simulink model "sm_car"  (R2026a)
settings: Solver=ode23t  StopTime=100  MaxStep=0.4  AbsTol=1e-3  EnableMultiTasking=on
PreLoadFcn:
  | % Due to usability issue in Repeating Sequence block
  | warning('off','Simulink:Masking:Invalid');
  | 
  | % Eliminate unnecessary warnings in inactive variants
  | % Warnings generated only if you click through inactive variant
  | warning('off','MATLAB:nonExistentField');
  | warning('off','Simulink:Parameters:BlkParamUndefined');
PostLoadFcn:
  | warning('off','sm:sli:setup:compile:LocalSolverNotSupported')
  | %sm_car_config_maneuver(bdroot,'WOT Braking');
  | sm_car_config_vehicle(bdroot,'false');
  | sm_car_config_logging(bdroot);
InitFcn:
  | sm_car_config_camera;
  | Vehicle = sm_car_vehcfg_checkConfig(Vehicle);
  | sm_car_check_tire_model(bdroot);
StartFcn:
  | tic;
StopFcn:
  | Elapsed_Sim_Time = toc;
  | % disp(['Elapsed Sim Time = ' num2str(Elapsed_Sim_Time)]);
undefined symbols (not defined in the file): Camera, Control, Driver, Maneuver, Pedal, Scene, Soft, Stiff, Visual, X, xy_data_car_side, Y, Z
libraries: sm_lib x207, simulink x21, nesl_utility x6, simulink_extras x4, slpidlib x1
(part 5 of 13)

== system sm_car/Driver/Closed Loop/Override ==
  "dist " : Inport
  "Obs " : Inport  Port=2
  None : Subsystem  VariantControl=None  mask(No Driver Override){override=Scene.Mallory_Park_Obstacle.Override}
      mask prompts: override "Override parameters (structure)"
      mask help: Driver commands are not overridden, regardless of inputs to subsystem.
  " Ovr" : Outport  VectorParamsAs1DForOutWhenUnconnected=off

== system sm_car/Driver/Closed Loop/Scopes ==
  <vx> : Inport
  Ref : Inport  Port=2
  CurPose : Inport  Port=3
  DrvBus : Inport  Port=4
  Bus Selector : BusSelector  OutputSignals=vTarget
  Bus Selector1 : BusSelector  OutputSignals=aSteerWheel,rAccelPedal,rBrakePedal
  Compare vx to Target : Scope  NumInputPorts=2
      settings: ActiveDisplayYMinimum=-4.79181  ActiveDisplayYMaximum=0.54534
  RefPose : Scope
      settings: ActiveDisplayYMinimum=-598.75829  ActiveDisplayYMaximum=469.37365
  Scope1 : Scope  NumInputPorts=3
      settings: ActiveDisplayYMinimum=-1.19495  ActiveDisplayYMaximum=0.13277  DataLoggingVariableName=ScopeData2
  wires:
  DrvBus/1 -> Bus Selector1/1
  Bus Selector1/1 -> Scope1/1  "<aSteerWheel>"
  Bus Selector1/2 -> Scope1/2  "<rAccelPedal>"
  <vx>/1 -> Compare vx to Target/1
  Bus Selector1/3 -> Scope1/3  "<rBrakePedal>"
  CurPose/1 -> RefPose/1
  Bus Selector/1 -> Compare vx to Target/2  "<vTarget>"
  Ref/1 -> Bus Selector/1

== system sm_car/Driver/Open Loop/Open Loop ==
  Bus Creator : BusCreator  Inputs=7
  Bus Creator5 : BusCreator  Inputs=4
  Constant : Constant  Value=10000
  Constant{1..6} (6 alike) : Constant  Value=0
  Input Sequence Accel Pedal : simulink/Sources/Repeating Sequence  rep_seq_t=Maneuver.Accel.t.Value  rep_seq_y=Maneuver.Accel.rPedal.Value
  Input Sequence Brake Pedal : simulink/Sources/Repeating Sequence  rep_seq_t=Maneuver.Brake.t.Value  rep_seq_y=Maneuver.Brake.rPedal.Value
  "Input Sequence Steering Wheel " : simulink/Sources/Repeating Sequence  rep_seq_t=Maneuver.Steer.t.Value  rep_seq_y=Maneuver.Steer.aWheel.Value
  DrvBus : Outport  VectorParamsAs1DForOutWhenUnconnected=off
  wires:
  Constant6/1 -> Bus Creator/7  "nLap"
  Constant/1 -> Bus Creator/1  "dist"
  Bus Creator/1 -> Bus Creator5/1  "Reference"
  Constant4/1 -> Bus Creator/5  "vTarget"
  Constant3/1 -> Bus Creator/4  "ayaw"
  Constant2/1 -> Bus Creator/3  "y"
  Constant5/1 -> Bus Creator/6  "latdev"
  Constant1/1 -> Bus Creator/2  "x"
  Input Sequence Accel Pedal/1 -> Bus Creator5/3  "rAccelPedal"
  "Input Sequence Steering Wheel "/1 -> Bus Creator5/2  "aSteerWheel"
  Input Sequence Brake Pedal/1 -> Bus Creator5/4  "rBrakePedal"
  Bus Creator5/1 -> DrvBus/1  "DrvBus"

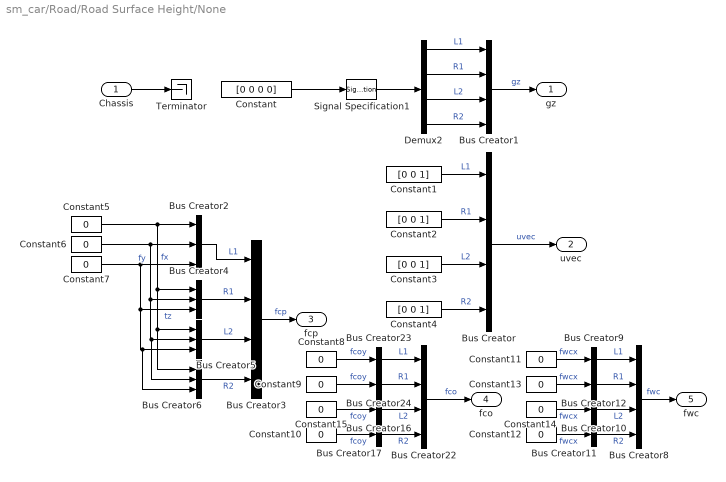
== system sm_car/Road/Road Surface Height/None ==
  Chassis : Inport
  Bus Creator{,1,3,8,22} (5 alike) : BusCreator  Inputs=4
  Bus Creator{9..12,16..17,23..24} (8 alike) : BusCreator  Inputs=1
  Bus Creator{2,4..6} (4 alike) : BusCreator  Inputs=3
  Constant : Constant  Value=[0 0 0 0]
  Constant{1..4} (4 alike) : Constant  Value=[0 0 1]
  Constant{5..15} (11 alike) : Constant  Value=0
  Demux2 : Demux
  Signal Specification1 : SignalSpecification  Unit=m
  Terminator : Terminator
  gz : Outport  VectorParamsAs1DForOutWhenUnconnected=off
  uvec : Outport  Port=2  VectorParamsAs1DForOutWhenUnconnected=off
  fcp : Outport  Port=3  VectorParamsAs1DForOutWhenUnconnected=off
  fco : Outport  Port=4  VectorParamsAs1DForOutWhenUnconnected=off
  fwc : Outport  Port=5  VectorParamsAs1DForOutWhenUnconnected=off
  wires:
  Bus Creator24/1 -> Bus Creator22/2  "R1"
  Constant13/1 -> Bus Creator12/1  "fwcx"
  Constant14/1 -> Bus Creator10/1  "fwcx"
  Constant12/1 -> Bus Creator11/1  "fwcx"
  Bus Creator12/1 -> Bus Creator8/2  "R1"
  Bus Creator10/1 -> Bus Creator8/3  "L2"
  Constant11/1 -> Bus Creator9/1  "fwcx"
  Bus Creator23/1 -> Bus Creator22/1  "L1"
  Bus Creator17/1 -> Bus Creator22/4  "R2"
  Constant10/1 -> Bus Creator17/1  "fcoy"
  Bus Creator9/1 -> Bus Creator8/1  "L1"
  Constant9/1 -> Bus Creator24/1  "fcoy"
  Bus Creator8/1 -> fwc/1  "fwc"
  Bus Creator22/1 -> fco/1  "fco"
  Constant15/1 -> Bus Creator16/1  "fcoy"
  Bus Creator16/1 -> Bus Creator22/3  "L2"
  Bus Creator11/1 -> Bus Creator8/4  "R2"
  Constant8/1 -> Bus Creator23/1  "fcoy"
  Bus Creator/1 -> uvec/1  "uvec"
  Constant4/1 -> Bus Creator/4  "R2"
  Constant1/1 -> Bus Creator/1  "L1"
  Constant2/1 -> Bus Creator/2  "R1"
  Constant3/1 -> Bus Creator/3  "L2"
  Demux2/3 -> Bus Creator1/3  "L2"
  Demux2/4 -> Bus Creator1/4  "R2"
  Demux2/2 -> Bus Creator1/2  "R1"
  Bus Creator1/1 -> gz/1  "gz"
  Signal Specification1/1 -> Demux2/1
  Demux2/1 -> Bus Creator1/1  "L1"
  Constant/1 -> Signal Specification1/1
  Chassis/1 -> Terminator/1
  Constant5/1 -> Bus Creator6/1, Bus Creator5/1, Bus Creator4/1, Bus Creator2/1  "fx"
  Constant6/1 -> Bus Creator6/2, Bus Creator5/2, Bus Creator4/2, Bus Creator2/2  "fy"
  Constant7/1 -> Bus Creator6/3, Bus Creator5/3, Bus Creator4/3, Bus Creator2/3  "tz"
  Bus Creator2/1 -> Bus Creator3/1  "L1"
  Bus Creator3/1 -> fcp/1  "fcp"
  Bus Creator4/1 -> Bus Creator3/2  "R1"
  Bus Creator5/1 -> Bus Creator3/3  "L2"
  Bus Creator6/1 -> Bus Creator3/4  "R2"

== system sm_car/Road/Surface Mu Scaling/Constant ==
  One : Constant  Value=scaleCoefficient  OutDataTypeStr=Inherit: Inherit via back propagation
  Scaling factors L1 : Subsystem  mask{LKX=1, LKY=1, LKYC=1, LTR=1, LKZC=1}
      mask prompts: LKX "longitudinal slip stiffness"; LKY "cornering stiffness"; LKYC "camber stiffness"; LTR "pneumatic trail"; LKZC "camber torque stiffness"
  Scaling factors L2 : Subsystem  mask{LKX=1, LKY=1, LKYC=1, LTR=1, LKZC=1}
      mask prompts: LKX "longitudinal slip stiffness"; LKY "cornering stiffness"; LKYC "camber stiffness"; LTR "pneumatic trail"; LKZC "camber torque stiffness"
  Scaling factors R1 : Subsystem  mask{LKX=1, LKY=1, LKYC=1, LTR=1, LKZC=1}
      mask prompts: LKX "longitudinal slip stiffness"; LKY "cornering stiffness"; LKYC "camber stiffness"; LTR "pneumatic trail"; LKZC "camber torque stiffness"
  Scaling factors R2 : Subsystem  mask{LKX=1, LKY=1, LKYC=1, LTR=1, LKZC=1}
      mask prompts: LKX "longitudinal slip stiffness"; LKY "cornering stiffness"; LKYC "camber stiffness"; LTR "pneumatic trail"; LKZC "camber torque stiffness"
  L1 : Outport  VectorParamsAs1DForOutWhenUnconnected=off
  R1 : Outport  Port=2  VectorParamsAs1DForOutWhenUnconnected=off
  L2 : Outport  Port=3  VectorParamsAs1DForOutWhenUnconnected=off
  R2 : Outport  Port=4  VectorParamsAs1DForOutWhenUnconnected=off
  wires:
  Scaling factors L1/1(scaling) -> L1/1  "TyreScalingL1"
  One/1 -> Scaling factors L1/1(muX), Scaling factors L1/2(muY), Scaling factors R1/1(muX), Scaling factors R1/2(muY), Scaling factors L2/1(muX), Scaling factors L2/2(muY), Scaling factors R2/1(muX), Scaling factors R2/2(muY)
  Scaling factors R1/1(scaling) -> R1/1  "TyreScalingR1"
  Scaling factors R2/1(scaling) -> R2/1  "TyreScalingR2"
  Scaling factors L2/1(scaling) -> L2/1  "TyreScalingL2"

== system sm_car/Visualization/Unreal/Animation Off ==
  xyz : Inport
  rpy : Inport  Port=2
  ws : Inport  Port=3
  aCamber : Inport  Port=4
  aSteerWheel : Inport  Port=5
  Terminator{,1..4} (5 alike) : Terminator
  wires:
  rpy/1 -> Terminator1/1
  aSteerWheel/1 -> Terminator4/1
  aCamber/1 -> Terminator3/1
  xyz/1 -> Terminator/1
  ws/1 -> Terminator2/1

== system sm_car/World/Mechanism Configuration/Constant Gravity ==
  MechanismConfiguration : sm_lib/Utilities/Mechanism Configuration  UniformGravity=Constant  GravityVector=GravityVector  GravityVectorUnits=m/s^2  LinearizationDelta=0.001  JointModeTransitionNonlinearIterations=2
  C : PMIOPort  Side=Right
  connections:
  MechanismConfiguration/RConn1 -- C/RConn1

== system sm_car/World/Scene/CRG Hockenheim ==
  Finish Line : Subsystem  mask{post_h=geometry.finish_line.post.height, post_r=geometry.finish_line.post.radius, line_w=geometry.finish_line.post.separation, post_clr=geometry.finish_line.post.clr, post_opc=geometry.finish_line.post.opc, offset_xyz=geometry.finish_line.offset.xyz, offset_yaw=geometry.finish_line.offset.yaw, offset_pitch=geometry.finish_line.offset.pitch, offset_roll=geometry.finish_line.offset.roll}
      mask prompts: post_h "Post Height (m)"; post_r "Post Radius (m)"; line_w "Post Separation (m)"; post_clr "Post Color [R G B] (0-1)"; post_opc "Post Opacity (0-1)"; offset_xyz "Line Offset [x y z] (m)"; offset_yaw "Line Orientation yaw (rad)"; offset_pitch "Line Orientation pitch (rad)"; offset_roll "Line Orientation roll (rad)"
  Ground : Ground
  STL Geometry Centerline : Subsystem  mask{stl_file=geometry.centerline.filename, stl_units=geometry.centerline.fileunits, stl_clr=geometry.centerline.clr, stl_opc=geometry.centerline.opc, stl_x=geometry.centerline.x, stl_y=geometry.centerline.y, stl_z=geometry.centerline.z, stl_yaw=geometry.centerline.yaw, stl_pitch=geometry.centerline.pitch, stl_roll=geometry.centerline.roll}
      mask prompts: stl_file "CAD File"; stl_units "Units"; stl_clr "Color [R G B]"; stl_opc "Opacity (0-1)"; stl_x "Offset x (m)"; stl_y "Offset y (m)"; stl_z "Offset z (m)"; stl_yaw "Offset yaw (rad)"; stl_pitch "Offset pitch (rad)"; stl_roll "Offset roll (rad)"
      mask init:
      | set_param([gcb '/Geometry'],'ExtGeomFileName',stl_file);
      | set_param([gcb '/Geometry'],'ExtGeomFileUnits',stl_units);
  STL Geometry Road : Subsystem  mask{stl_file=geometry.filename, stl_units=geometry.fileunits, stl_clr=geometry.clr, stl_opc=geometry.opc, stl_x=geometry.x, stl_y=geometry.y, stl_z=geometry.z, stl_yaw=geometry.yaw, stl_pitch=geometry.pitch, stl_roll=geometry.roll}
      mask prompts: stl_file "CAD File"; stl_units "Units"; stl_clr "Color [R G B]"; stl_opc "Opacity (0-1)"; stl_x "Offset x (m)"; stl_y "Offset y (m)"; stl_z "Offset z (m)"; stl_yaw "Offset yaw (rad)"; stl_pitch "Offset pitch (rad)"; stl_roll "Offset roll (rad)"
      mask init:
      | set_param([gcb '/Geometry'],'ExtGeomFileName',stl_file);
      | set_param([gcb '/Geometry'],'ExtGeomFileUnits',stl_units);
  W : PMIOPort  Side=Left
  Obs : Outport  VectorParamsAs1DForOutWhenUnconnected=off
  wires:
  Ground/1 -> Obs/1
  connections:
  STL Geometry Centerline/RConn1 -- Finish Line/LConn1 -- W/RConn1 -- STL Geometry Road/RConn1

== system sm_car/World/Scene/CRG Hockenheim F ==
  Finish Line : Subsystem  mask{post_h=geometry.finish_line.post.height, post_r=geometry.finish_line.post.radius, line_w=geometry.finish_line.post.separation, post_clr=geometry.finish_line.post.clr, post_opc=geometry.finish_line.post.opc, offset_xyz=geometry.finish_line.offset.xyz, offset_yaw=geometry.finish_line.offset.yaw, offset_pitch=geometry.finish_line.offset.pitch, offset_roll=geometry.finish_line.offset.roll}
      mask prompts: post_h "Post Height (m)"; post_r "Post Radius (m)"; line_w "Post Separation (m)"; post_clr "Post Color [R G B] (0-1)"; post_opc "Post Opacity (0-1)"; offset_xyz "Line Offset [x y z] (m)"; offset_yaw "Line Orientation yaw (rad)"; offset_pitch "Line Orientation pitch (rad)"; offset_roll "Line Orientation roll (rad)"
  Ground : Ground
  STL Geometry Centerline : Subsystem  mask{stl_file=geometry.centerline.filename, stl_units=geometry.centerline.fileunits, stl_clr=geometry.centerline.clr, stl_opc=geometry.centerline.opc, stl_x=geometry.centerline.x, stl_y=geometry.centerline.y, stl_z=geometry.centerline.z, stl_yaw=geometry.centerline.yaw, stl_pitch=geometry.centerline.pitch, stl_roll=geometry.centerline.roll}
      mask prompts: stl_file "CAD File"; stl_units "Units"; stl_clr "Color [R G B]"; stl_opc "Opacity (0-1)"; stl_x "Offset x (m)"; stl_y "Offset y (m)"; stl_z "Offset z (m)"; stl_yaw "Offset yaw (rad)"; stl_pitch "Offset pitch (rad)"; stl_roll "Offset roll (rad)"
      mask init:
      | set_param([gcb '/Geometry'],'ExtGeomFileName',stl_file);
      | set_param([gcb '/Geometry'],'ExtGeomFileUnits',stl_units);
  STL Geometry Road : Subsystem  mask{stl_file=geometry.filename, stl_units=geometry.fileunits, stl_clr=geometry.clr, stl_opc=geometry.opc, stl_x=geometry.x, stl_y=geometry.y, stl_z=geometry.z, stl_yaw=geometry.yaw, stl_pitch=geometry.pitch, stl_roll=geometry.roll}
      mask prompts: stl_file "CAD File"; stl_units "Units"; stl_clr "Color [R G B]"; stl_opc "Opacity (0-1)"; stl_x "Offset x (m)"; stl_y "Offset y (m)"; stl_z "Offset z (m)"; stl_yaw "Offset yaw (rad)"; stl_pitch "Offset pitch (rad)"; stl_roll "Offset roll (rad)"
      mask init:
      | set_param([gcb '/Geometry'],'ExtGeomFileName',stl_file);
      | set_param([gcb '/Geometry'],'ExtGeomFileUnits',stl_units);
  W : PMIOPort  Side=Left
  Obs : Outport  VectorParamsAs1DForOutWhenUnconnected=off
  wires:
  Ground/1 -> Obs/1
  connections:
  STL Geometry Centerline/RConn1 -- Finish Line/LConn1 -- W/RConn1 -- STL Geometry Road/RConn1

== system sm_car/World/Scene/Plane Grid ==
  Grid : Subsystem  mask{grid_x=plane.l, grid_y=plane.w, grid_z=plane.h, grid_line_width=grid.line_width, grid_num_sq_x=grid.num_sqrs_x, grid_num_sq_y=grid.num_sqrs_y, grid_clr=grid.clr, grid_opc=grid.opc}
      mask prompts: grid_x "Length (m) (Global x)"; grid_y "Width (m) (Global y)"; grid_z "Depth (m) (Global z)"; grid_line_width "Line width (m)"; grid_num_sq_x "Number of squares in x"; grid_num_sq_y "Number of squares in y"; grid_clr "Color [RGB]"; grid_opc "Opacity (0-1)"
      mask init:
      | % Derived parameters - for two perpendicular grids with num_sq-by-1 holes
      | % **Note, not num_sq_x by num_sq_y holes - better render speed with
      | % separate meshes for x and y.
      | 
      | hole_lx = (grid_x-(grid_line_width*(grid_num_sq_x+1)))/grid_num_sq_x;
      | hole_wx = (grid_y-(grid_line_width*(1+1)))/1;
      | 
      | hole_ly = (grid_y-(grid_line_width*(grid_num_sq_y+1)))/grid_num_sq_y;
      | hole_wy = (grid_x-(grid_line_width*(1+1)))/1;
  Ground : Ground
  Ground Plane : Subsystem  mask{gp_l=plane.l, gp_w=plane.w, gp_h=plane.h, gp_clr=plane.clr, gp_opc=plane.opc}
      mask prompts: gp_l "Length (m) (Global  x)"; gp_w "Width (m) (Global  y)"; gp_h "Depth (m) (Global z)"; gp_clr "Color [R G B]"; gp_opc "Opacity (0-1)"
  Transform Plane : sm_lib/Frames and Transforms/Rigid Transform  RotationMethod=None  FollAlignAxisA=+X  BaseAlignAxisA=+Y  FollAlignAxisB=+Y  BaseAlignAxisB=+Z  RotationStandardAxis=+Z  RotationAngle=0.0  RotationAngleUnits=deg  RotationArbitraryAxis=[0 0 1]  RotationSequenceAxes=FollowerAxes  RotationSequence=XYX  RotationSequenceAngles=[0 0 0]  RotationSequenceAnglesUnits=deg  RotationMatrix=[1 0 0; 0 1 0; 0 0 1]  Quaternion=[1 0 0 0]  TranslationMethod=Cartesian  TranslationCartesianOffset=[plane.x plane.y plane.z]  TranslationCartesianOffsetUnits=m  TranslationStandardAxis=+Z  TranslationStandardOffset=0  TranslationStandardOffsetUnits=m  TranslationROffset=0  TranslationROffsetUnits=m  TranslationThetaOffset=0  TranslationThetaOffsetUnits=deg  TranslationZOffset=0  TranslationZOffsetUnits=m
  W : PMIOPort  Side=Left
  Obs : Outport  VectorParamsAs1DForOutWhenUnconnected=off
  wires:
  Ground/1 -> Obs/1
  connections:
  Ground Plane/RConn1 -- Transform Plane/RConn1 -- Grid/LConn1
  Transform Plane/LConn1 -- W/RConn1

== system sm_car/World/Scene/Skidpad ==
  Circle Inner L : Subsystem  mask{circ_d=circ_in.d, circ_a1=-180, circ_a2=180, circ_w=circ_in.w, circ_h=circ_in.h, circ_clr=circ_in.clr, circ_opc=circ_in.opc}
      mask prompts: circ_d "Circle Diameter (m)"; circ_a1 "Start Angle (deg)"; circ_a2 "Finish Angle (deg)"; circ_w "Stripe Width (m)"; circ_h "Stripe Height (m)"; circ_clr "Color [RGB]"; circ_opc "Opacity (0-1)"
      mask init:
      | xy_data_circ = Extr_Data_Ring(...
      |     circ_d/2+circ_w/2,circ_d/2-circ_w/2,circ_a1, circ_a2);
  Circle Inner R : Subsystem  mask{circ_d=circ_in.d, circ_a1=-180, circ_a2=180, circ_w=circ_in.w, circ_h=circ_in.h, circ_clr=circ_in.clr, circ_opc=circ_in.opc}
      mask prompts: circ_d "Circle Diameter (m)"; circ_a1 "Start Angle (deg)"; circ_a2 "Finish Angle (deg)"; circ_w "Stripe Width (m)"; circ_h "Stripe Height (m)"; circ_clr "Color [RGB]"; circ_opc "Opacity (0-1)"
      mask init:
      | xy_data_circ = Extr_Data_Ring(...
      |     circ_d/2+circ_w/2,circ_d/2-circ_w/2,circ_a1, circ_a2);
  Circle Outer L : Subsystem  mask{circ_d=circ_out.d, circ_a1=circ_out.ang1, circ_a2=circ_out.ang2, circ_w=circ_out.w, circ_h=circ_out.h, circ_clr=circ_out.clr, circ_opc=circ_out.opc}
      mask prompts: circ_d "Circle Diameter (m)"; circ_a1 "Start Angle (deg)"; circ_a2 "Finish Angle (deg)"; circ_w "Stripe Width (m)"; circ_h "Stripe Height (m)"; circ_clr "Color [RGB]"; circ_opc "Opacity (0-1)"
      mask init:
      | xy_data_circ = Extr_Data_Ring(...
      |     circ_d/2+circ_w/2,circ_d/2-circ_w/2,circ_a1, circ_a2);
  Circle Outer R : Subsystem  mask{circ_d=circ_out.d, circ_a1=circ_out.ang1, circ_a2=circ_out.ang2, circ_w=circ_out.w, circ_h=circ_out.h, circ_clr=circ_out.clr, circ_opc=circ_out.opc}
      mask prompts: circ_d "Circle Diameter (m)"; circ_a1 "Start Angle (deg)"; circ_a2 "Finish Angle (deg)"; circ_w "Stripe Width (m)"; circ_h "Stripe Height (m)"; circ_clr "Color [RGB]"; circ_opc "Opacity (0-1)"
      mask init:
      | xy_data_circ = Extr_Data_Ring(...
      |     circ_d/2+circ_w/2,circ_d/2-circ_w/2,circ_a1, circ_a2);
  Ground : Ground
  Ground Plane : Subsystem  mask{gp_l=plane.l, gp_w=plane.w, gp_h=plane.h, gp_clr=plane.clr, gp_opc=plane.opc}
      mask prompts: gp_l "Length (m) (Global  x)"; gp_w "Width (m) (Global  y)"; gp_h "Depth (m) (Global z)"; gp_clr "Color [R G B]"; gp_opc "Opacity (0-1)"
  Transform Circle L : sm_lib/Frames and Transforms/Rigid Transform  RotationMethod=None  FollAlignAxisA=+X  BaseAlignAxisA=+Y  FollAlignAxisB=+Y  BaseAlignAxisB=+Z  RotationStandardAxis=+Z  RotationAngle=0.0  RotationAngleUnits=deg  RotationArbitraryAxis=[0 0 1]  RotationSequenceAxes=FollowerAxes  RotationSequence=XYX  RotationSequenceAngles=[0 0 0]  RotationSequenceAnglesUnits=deg  RotationMatrix=[1 0 0; 0 1 0; 0 0 1]  Quaternion=[1 0 0 0]  TranslationMethod=Cartesian  TranslationCartesianOffset=[0 circ_in.sep/2 0]  TranslationCartesianOffsetUnits=m  TranslationStandardAxis=+Z  TranslationStandardOffset=0  TranslationStandardOffsetUnits=m  TranslationROffset=0  TranslationROffsetUnits=m  TranslationThetaOffset=0  TranslationThetaOffsetUnits=deg  TranslationZOffset=0  TranslationZOffsetUnits=m
  Transform Circle R : sm_lib/Frames and Transforms/Rigid Transform  RotationMethod=None  FollAlignAxisA=+X  BaseAlignAxisA=+Y  FollAlignAxisB=+Y  BaseAlignAxisB=+Z  RotationStandardAxis=+Z  RotationAngle=0.0  RotationAngleUnits=deg  RotationArbitraryAxis=[0 0 1]  RotationSequenceAxes=FollowerAxes  RotationSequence=XYX  RotationSequenceAngles=[0 0 0]  RotationSequenceAnglesUnits=deg  RotationMatrix=[1 0 0; 0 1 0; 0 0 1]  Quaternion=[1 0 0 0]  TranslationMethod=Cartesian  TranslationCartesianOffset=[0 -circ_in.sep/2 0]  TranslationCartesianOffsetUnits=m  TranslationStandardAxis=+Z  TranslationStandardOffset=0  TranslationStandardOffsetUnits=m  TranslationROffset=0  TranslationROffsetUnits=m  TranslationThetaOffset=0  TranslationThetaOffsetUnits=deg  TranslationZOffset=0  TranslationZOffsetUnits=m
  Transform Orient OuterL : sm_lib/Frames and Transforms/Rigid Transform  RotationMethod=StandardAxis  FollAlignAxisA=+X  BaseAlignAxisA=+Y  FollAlignAxisB=+Y  BaseAlignAxisB=+Z  RotationStandardAxis=+Z  RotationAngle=90  RotationAngleUnits=deg  RotationArbitraryAxis=[0 0 1]  RotationSequenceAxes=FollowerAxes  RotationSequence=XYX  RotationSequenceAngles=[0 0 0]  RotationSequenceAnglesUnits=deg  RotationMatrix=[1 0 0; 0 1 0; 0 0 1]  Quaternion=[1 0 0 0]  TranslationMethod=None  TranslationCartesianOffset=[0 0 0]  TranslationCartesianOffsetUnits=m  TranslationStandardAxis=+Z  TranslationStandardOffset=0  TranslationStandardOffsetUnits=m  TranslationROffset=0  TranslationROffsetUnits=m  TranslationThetaOffset=0  TranslationThetaOffsetUnits=deg  TranslationZOffset=0  TranslationZOffsetUnits=m
  Transform Orient OuterR : sm_lib/Frames and Transforms/Rigid Transform  RotationMethod=StandardAxis  FollAlignAxisA=+X  BaseAlignAxisA=+Y  FollAlignAxisB=+Y  BaseAlignAxisB=+Z  RotationStandardAxis=+Z  RotationAngle=-90  RotationAngleUnits=deg  RotationArbitraryAxis=[0 0 1]  RotationSequenceAxes=FollowerAxes  RotationSequence=XYX  RotationSequenceAngles=[0 0 0]  RotationSequenceAnglesUnits=deg  RotationMatrix=[1 0 0; 0 1 0; 0 0 1]  Quaternion=[1 0 0 0]  TranslationMethod=None  TranslationCartesianOffset=[0 0 0]  TranslationCartesianOffsetUnits=m  TranslationStandardAxis=+Z  TranslationStandardOffset=0  TranslationStandardOffsetUnits=m  TranslationROffset=0  TranslationROffsetUnits=m  TranslationThetaOffset=0  TranslationThetaOffsetUnits=deg  TranslationZOffset=0  TranslationZOffsetUnits=m
  Transform Plane : sm_lib/Frames and Transforms/Rigid Transform  RotationMethod=None  FollAlignAxisA=+X  BaseAlignAxisA=+Y  FollAlignAxisB=+Y  BaseAlignAxisB=+Z  RotationStandardAxis=+Z  RotationAngle=0.0  RotationAngleUnits=deg  RotationArbitraryAxis=[0 0 1]  RotationSequenceAxes=FollowerAxes  RotationSequence=XYX  RotationSequenceAngles=[0 0 0]  RotationSequenceAnglesUnits=deg  RotationMatrix=[1 0 0; 0 1 0; 0 0 1]  Quaternion=[1 0 0 0]  TranslationMethod=Cartesian  TranslationCartesianOffset=[plane.x plane.y plane.z]  TranslationCartesianOffsetUnits=m  TranslationStandardAxis=+Z  TranslationStandardOffset=0  TranslationStandardOffsetUnits=m  TranslationROffset=0  TranslationROffsetUnits=m  TranslationThetaOffset=0  TranslationThetaOffsetUnits=deg  TranslationZOffset=0  TranslationZOffsetUnits=m
  W : PMIOPort  Side=Left
  Obs : Outport  VectorParamsAs1DForOutWhenUnconnected=off
  wires:
  Ground/1 -> Obs/1
  connections:
  Circle Outer L/RConn1 -- Transform Orient OuterL/RConn1
  Circle Outer R/RConn1 -- Transform Orient OuterR/RConn1
  Circle Inner R/RConn1 -- Transform Circle R/RConn1 -- Transform Orient OuterR/LConn1
  Transform Plane/RConn1 -- Ground Plane/RConn1
  Transform Circle L/LConn1 -- W/RConn1 -- Transform Plane/LConn1 -- Transform Circle R/LConn1
  Circle Inner L/RConn1 -- Transform Circle L/RConn1 -- Transform Orient OuterL/LConn1

== system sm_car/World/Visuals/Off ==
  Reference Frame : sm_lib/Frames and Transforms/Reference Frame
  W : PMIOPort  Side=Left
  connections:
  Reference Frame/RConn1 -- W/RConn1

== system sm_car/Controller/Default/Brake Control/Pedal ==
  rBrakePedal : Inport
  VehBus : Inport  Port=2
  Apply{,1..3} (4 alike) : Constant  Value=[0 1]
  Bus Creator : BusCreator  Inputs=1
  Bus Creator1 : BusCreator  Inputs=4
  Terminator : Terminator
  Terminator1 : Terminator
  Brakes : Outport  VectorParamsAs1DForOutWhenUnconnected=off
  wires:
  rBrakePedal/1 -> Terminator1/1
  Apply3/1 -> Bus Creator1/4  "R2"
  Apply2/1 -> Bus Creator1/3  "L2"
  Apply1/1 -> Bus Creator1/2  "R1"
  Apply/1 -> Bus Creator1/1  "L1"
  Bus Creator1/1 -> Bus Creator/1  "Valves"
  VehBus/1 -> Terminator/1
  Bus Creator/1 -> Brakes/1  "Brakes"

== system sm_car/Controller/Default/Damper Control/Damper Control A1 ==
  mL : Inport
  mR : Inport  Port=2
  Inp : Inport  Port=3
  None : Subsystem  VariantControl=None
  L : Outport
  R : Outport  Port=2

== system sm_car/Controller/Default/Damper Control/Damper Control A2 ==
  mL : Inport
  mR : Inport  Port=2
  Inp : Inport  Port=3
  None : Subsystem  VariantControl=None
  L : Outport
  R : Outport  Port=2

== system sm_car/Controller/Default/Spring Control/Spring Control A1 ==
  mL : Inport
  mR : Inport  Port=2
  Inp : Inport  Port=3
  Hydropneumatic : Subsystem  VariantControl=Hydropneumatic  mask{popup_gas_spring=Soft}
      mask prompts: popup_gas_spring "Gas Spring"
      mask init:
      | bh = gcb;
      | popup_gas_spring_str = get_param(bh,'popup_gas_spring');
      | 
      | if(strcmp(popup_gas_spring_str,'Stiff'))
      |     soft_suspension = 0;
      | elseif(strcmp(popup_gas_spring_str,'Soft'))
      |     soft_suspension = 1;
      | end
      mask TypeOptions popup_gas_spring: Stiff | Soft
  None : Subsystem  VariantControl=None
  L : Outport  VectorParamsAs1DForOutWhenUnconnected=off
  R : Outport  Port=2  VectorParamsAs1DForOutWhenUnconnected=off

== system sm_car/Controller/Default/Spring Control/Spring Control A2 ==
  mL : Inport
  mR : Inport  Port=2
  Inp : Inport  Port=3
  Hydropneumatic : Subsystem  VariantControl=Hydropneumatic  mask{popup_gas_spring=Soft}
      mask prompts: popup_gas_spring "Gas Spring"
      mask init: same as sm_car/Controller/Default/Spring Control/Spring Control A1/Hydropneumatic
      mask TypeOptions popup_gas_spring: Stiff | Soft
  None : Subsystem  VariantControl=None
  L : Outport  VectorParamsAs1DForOutWhenUnconnected=off
  R : Outport  Port=2  VectorParamsAs1DForOutWhenUnconnected=off

== system sm_car/Controller/Default/Susp/Steer Axle 1 ==
  note: Example Steer by Wire algorithm.
      | Used by steering models where rack position
      | and steering wheel angle inputs are both used.
  aSteerWheel : Inport
  vx : Inport  Port=2
  Bus Creator4 : BusCreator  Inputs=2
  Product1 : Product
  Transfer Fcn (with initial states)1 : simulink_extras/Additional Linear/Transfer Fcn (with initial states)  N=[1]  D="[1/Steer.fActuatorCutoff.Value  1]"  X0=-1
  Vehicle Speed to Ratio Scale : Lookup_n-D  NumberOfTableDimensions=1  BreakpointsForDimension1=Control.Default.Steer.Ratio_Scale.vVehicle.Value  Table=Control.Default.Steer.Ratio_Scale.n.Value  InternalRulePriority=Speed  RndMeth=Simplest
  Wheel Angle to Steer Ratio : Lookup_n-D  NumberOfTableDimensions=1  BreakpointsForDimension1=Control.Default.Steer.Ratio_Table.aWheel.Value  Table=Control.Default.Steer.Ratio_Table.xRack.Value  InternalRulePriority=Speed  RndMeth=Simplest
  Steer : Outport  VectorParamsAs1DForOutWhenUnconnected=off
  wires:
  Vehicle Speed to Ratio Scale/1 -> Product1/1  "nRatioScale"
  Transfer Fcn (with initial states)1/1 -> Vehicle Speed to Ratio Scale/1
  aSteerWheel/1 -> Wheel Angle to Steer Ratio/1, Bus Creator4/2  "aSteerWheel"
  Wheel Angle to Steer Ratio/1 -> Product1/2  "xRack"
  Product1/1 -> Bus Creator4/1  "xRack"
  vx/1 -> Transfer Fcn (with initial states)1/1
  Bus Creator4/1 -> Steer/1  "Steer"

== system sm_car/Controller/Default/Susp/Steer Axle 2 ==
  note: Example rear steer algorithm
      | Rack position is based on steering wheel angle
      | and is scaled based on vehicle speed.
  aSteerWheel : Inport
  vx : Inport  Port=2
  1-D Lookup Table : Lookup_n-D  NumberOfTableDimensions=1  BreakpointsForDimension1=Steer.Gain.vVehicle.Value  Table=Steer.Gain.n.Value  InterpMethod=Linear Lagrange  InternalRulePriority=Speed  RndMeth=Simplest
  Bus Creator2 : BusCreator  Inputs=2
  Filter : simulink_extras/Additional Linear/Transfer Fcn (with initial states)  N=[1]  D="[1/Steer.fActuatorCutoff.Value  1]"  X0=-1
  Gain : Gain  Gain=3.6
  Gain1 : Gain  Gain=Steer.Gain.nRearAct.Value
  Product : Product
  Saturation : Saturate  UpperLimit=Steer.Limits.aUpper.Value  LowerLimit=Steer.Limits.aLower.Value  LinearizeAsGain=off  ZeroCross=off
  Steer : Outport
  wires:
  aSteerWheel/1 -> Product/1
  Gain/1 -> 1-D Lookup Table/1
  Bus Creator2/1 -> Steer/1  "Steer"
  Saturation/1 -> Bus Creator2/1, Gain1/1  "aSteerWheel"
  Product/1 -> Saturation/1
  Filter/1 -> Product/2
  Gain1/1 -> Bus Creator2/2  "xSteerActuator"
  1-D Lookup Table/1 -> Filter/1
  vx/1 -> Gain/1

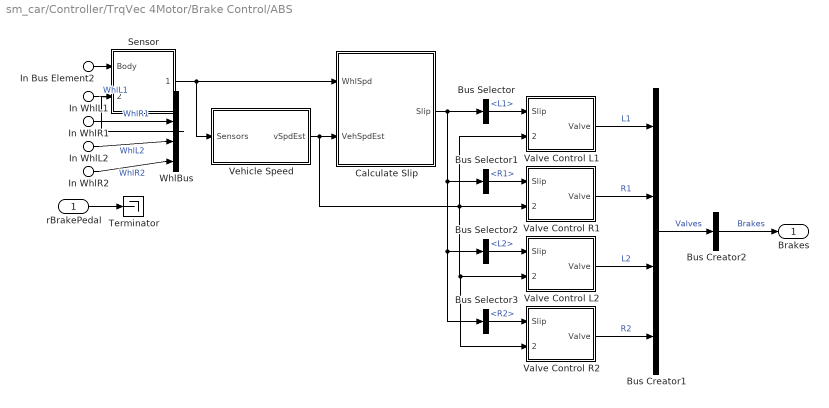
== system sm_car/Controller/TrqVec 4Motor/Brake Control/ABS ==
  rBrakePedal : Inport
  In Bus Element2 : Inport  Port=2  PortName=VehBus  Element=Body.CG
  In WhlL1 : Inport  Port=2  PortName=VehBus  Element=WhlL1
  In WhlR1 : Inport  Port=2  PortName=VehBus  Element=WhlR1
  In WhlL2 : Inport  Port=2  PortName=VehBus  Element=WhlL2
  In WhlR2 : Inport  Port=2  PortName=VehBus  Element=WhlR2
  Bus Creator1 : BusCreator  Inputs=4
  Bus Creator2 : BusCreator  Inputs=1
  Bus Selector : BusSelector  OutputSignals=L1
  Bus Selector1 : BusSelector  OutputSignals=R1
  Bus Selector2 : BusSelector  OutputSignals=L2
  Bus Selector3 : BusSelector  OutputSignals=R2
  Calculate Slip : Subsystem
  Sensor : Subsystem
  Terminator : Terminator
  Valve Control L1 : Subsystem
  Valve Control L2 : Subsystem
  Valve Control R1 : Subsystem
  Valve Control R2 : Subsystem
  Vehicle Speed : Subsystem
  WhlBus : BusCreator  Inputs=4
  Brakes : Outport  VectorParamsAs1DForOutWhenUnconnected=off
  wires:
  rBrakePedal/1 -> Terminator/1
  Vehicle Speed/1(vSpdEst) -> Valve Control R2/2(vSpdEst), Valve Control L2/2(vSpdEst), Valve Control R1/2(vSpdEst), Valve Control L1/2(vSpdEst), Calculate Slip/2(VehSpdEst)
  Sensor/1(GroundSpd) -> Vehicle Speed/1(Sensors), Calculate Slip/1(WhlSpd)
  Bus Creator1/1 -> Bus Creator2/1  "Valves"
  Bus Selector2/1 -> Valve Control L2/1(Slip)  "<L2>"
  Valve Control R1/1(Valve) -> Bus Creator1/2  "R1"
  Valve Control R2/1(Valve) -> Bus Creator1/4  "R2"
  Valve Control L2/1(Valve) -> Bus Creator1/3  "L2"
  Bus Selector3/1 -> Valve Control R2/1(Slip)  "<R2>"
  Bus Selector/1 -> Valve Control L1/1(Slip)  "<L1>"
  Calculate Slip/1(Slip) -> Bus Selector3/1, Bus Selector2/1, Bus Selector1/1, Bus Selector/1
  Valve Control L1/1(Valve) -> Bus Creator1/1  "L1"
  Bus Selector1/1 -> Valve Control R1/1(Slip)  "<R1>"
  Bus Creator2/1 -> Brakes/1  "Brakes"
  In Bus Element2/1 -> Sensor/1(Body)
  In WhlL1/1 -> WhlBus/1  "WhlL1"
  In WhlR1/1 -> WhlBus/2  "WhlR1"
  In WhlL2/1 -> WhlBus/3  "WhlL2"
  In WhlR2/1 -> WhlBus/4  "WhlR2"
  WhlBus/1 -> Sensor/2(WhlSpd)

== system sm_car/Controller/TrqVec 4Motor/Brake Control/Pedal ==
  rBrakePedal : Inport
  VehBus : Inport  Port=2
  Apply{,1..3} (4 alike) : Constant  Value=[0 1]
  Bus Creator : BusCreator  Inputs=1
  Bus Creator1 : BusCreator  Inputs=4
  Terminator : Terminator
  Terminator1 : Terminator
  Brakes : Outport  VectorParamsAs1DForOutWhenUnconnected=off
  wires:
  rBrakePedal/1 -> Terminator1/1
  Apply3/1 -> Bus Creator1/4  "R2"
  Apply2/1 -> Bus Creator1/3  "L2"
  Apply1/1 -> Bus Creator1/2  "R1"
  Apply/1 -> Bus Creator1/1  "L1"
  Bus Creator1/1 -> Bus Creator/1  "Valves"
  VehBus/1 -> Terminator/1
  Bus Creator/1 -> Brakes/1  "Brakes"

== system sm_car/Controller/TrqVec 4Motor/Brake Control/Pressure ==
  rBrakePedal : Inport
  VehBus : Inport  Port=2
  Bus Creator : BusCreator  Inputs=4
  Gain : Gain  Gain=Vehicle.Brakes.Front.Caliper.pMax.Value
  Gain1 : Gain  Gain=Vehicle.Brakes.Front.Caliper.pMax.Value
  Gain2 : Gain  Gain=Vehicle.Brakes.Rear.Caliper.pMax.Value
  Gain3 : Gain  Gain=Vehicle.Brakes.Rear.Caliper.pMax.Value
  Terminator : Terminator
  Brakes : Outport  VectorParamsAs1DForOutWhenUnconnected=off
  wires:
  rBrakePedal/1 -> Gain/1, Gain1/1, Gain3/1, Gain2/1
  VehBus/1 -> Terminator/1
  Bus Creator/1 -> Brakes/1  "Brakes"
  Gain/1 -> Bus Creator/1  "pBrakeL1"
  Gain1/1 -> Bus Creator/2  "pBrakeR1"
  Gain2/1 -> Bus Creator/3  "pBrakeL2"
  Gain3/1 -> Bus Creator/4  "pBrakeR2"

== system sm_car/Controller/TrqVec 4Motor/Damper Control/Damper Control A1 ==
  mL : Inport
  mR : Inport  Port=2
  Inp : Inport  Port=3
  Coefficient : Subsystem  VariantControl=Coefficient  mask(Control Law for Damper Coefficient){b_A1=ControlDamper.tFilt, brkPts_dim1_A1=ControlDamper.vDamperd, brkPts_dim2_A1=ControlDamper.iControl, Table_A1=ControlDamper.dDamper}
      mask prompts: b_A1 "Filter time constant (sec)"; brkPts_dim1_A1 "Damper Speed [1xm] (m/s)"; brkPts_dim2_A1 "Input 2 [1xn] (1)"; Table_A1 "Damper Coefficient [mxn] (N/(m/s))"
      mask help: Determines damping coefficient based on damper speed and a second input signal.
      mask TypeOptions b_A1: Filter/b
      mask TypeOptions brkPts_dim1_A1: Lookup Table Coeff/BreakpointsForDimension1
      mask TypeOptions brkPts_dim2_A1: Lookup Table Coeff/BreakpointsForDimension2
      mask TypeOptions Table_A1: Lookup Table Coeff/Table
      mask DialogControl cont_axle1 Prompt: Axle 1
  Force : Subsystem  VariantControl=Force  mask(Control Law for Damper Force){b_A1=ControlDamper.tFilt, brkPts_dim1_A1=ControlDamper.vDamperf, brkPts_dim2_A1=ControlDamper.iControl, Table_A1=ControlDamper.fDamper}
      mask prompts: b_A1 "Filter time constant (sec)"; brkPts_dim1_A1 "Damper Speed [1xm] (m/s)"; brkPts_dim2_A1 "Input 2 [1xn] (1)"; Table_A1 "Damper Force [mxn] (N)"
      mask help: Determines damping force based on damper speed and a second input signal.
      mask TypeOptions b_A1: Filter/b
      mask TypeOptions brkPts_dim1_A1: Lookup Table A1/BreakpointsForDimension1
      mask TypeOptions brkPts_dim2_A1: Lookup Table A1/BreakpointsForDimension2
      mask TypeOptions Table_A1: Lookup Table A1/Table
      mask DialogControl cont_axle1 Prompt: Axle 1
  None : Subsystem  VariantControl=None
  L : Outport
  R : Outport  Port=2

== system sm_car/Controller/TrqVec 4Motor/Damper Control/Damper Control A2 ==
  mL : Inport
  mR : Inport  Port=2
  Inp : Inport  Port=3
  Coefficient : Subsystem  VariantControl=Coefficient  mask(Control Law for Damper Coefficient){b_A1=ControlDamper.tFilt, brkPts_dim1_A1=ControlDamper.vDamperd, brkPts_dim2_A1=ControlDamper.iControl, Table_A1=ControlDamper.dDamper}
      mask prompts: b_A1 "Filter time constant (sec)"; brkPts_dim1_A1 "Damper Speed [1xm] (m/s)"; brkPts_dim2_A1 "Input 2 [1xn] (1)"; Table_A1 "Damper Coefficient [mxn] (N/(m/s))"
      mask help: Determines damping coefficient based on damper speed and a second input signal.
      mask TypeOptions b_A1: Filter/b
      mask TypeOptions brkPts_dim1_A1: Lookup Table Coeff/BreakpointsForDimension1
      mask TypeOptions brkPts_dim2_A1: Lookup Table Coeff/BreakpointsForDimension2
      mask TypeOptions Table_A1: Lookup Table Coeff/Table
      mask DialogControl cont_axle1 Prompt: Axle 1
  Force : Subsystem  VariantControl=Force  mask(Control Law for Damper Force){b_A1=ControlDamper.tFilt, brkPts_dim1_A1=ControlDamper.vDamperf, brkPts_dim2_A1=ControlDamper.iControl, Table_A1=ControlDamper.fDamper}
      mask prompts: b_A1 "Filter time constant (sec)"; brkPts_dim1_A1 "Damper Speed [1xm] (m/s)"; brkPts_dim2_A1 "Input 2 [1xn] (1)"; Table_A1 "Damper Force [mxn] (N)"
      mask help: Determines damping force based on damper speed and a second input signal.
      mask TypeOptions b_A1: Filter/b
      mask TypeOptions brkPts_dim1_A1: Lookup Table A1/BreakpointsForDimension1
      mask TypeOptions brkPts_dim2_A1: Lookup Table A1/BreakpointsForDimension2
      mask TypeOptions Table_A1: Lookup Table A1/Table
      mask DialogControl cont_axle1 Prompt: Axle 1
  None : Subsystem  VariantControl=None
  L : Outport
  R : Outport  Port=2

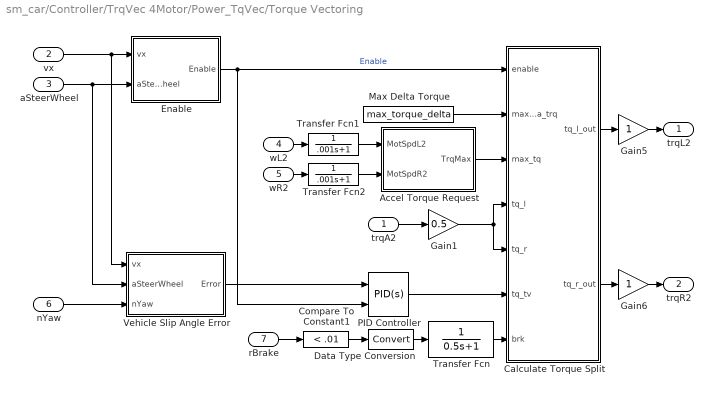
== system sm_car/Controller/TrqVec 4Motor/Power_TqVec/Torque Vectoring ==
  trqA2 : Inport
  vx : Inport  Port=2
  aSteerWheel : Inport  Port=3
  wL2 : Inport  Port=4
  wR2 : Inport  Port=5
  nYaw : Inport  Port=6
  rBrake : Inport  Port=7
  Accel Torque Request : Subsystem
  Calculate Torque Split : MATLAB Function  TreatAsAtomicUnit=on
  Compare To Constant1 : simulink/Logic and Bit Operations/Compare To Constant  relop=<  const=.01  OutDataTypeStr=boolean
  Data Type Conversion : DataTypeConversion  SaturateOnIntegerOverflow=off  RndMeth=Floor
  Enable : Subsystem
  Gain1 : Gain  Gain=0.5
  Gain5 : Gain
  Gain6 : Gain
  Max Delta Torque : Constant  Value=max_torque_delta
  PID Controller : slpidlib/PID Controller  Controller=PID  Form=Parallel  TimeDomain=Continuous-time  UseExternalTs=off  SampleTime=-1  IntegratorMethod=Forward Euler  FilterMethod=Forward Euler  ControllerParametersSource=internal  P=P  I=I  UseKiTs=off  D=0  UseExternalDerivativeSource=off  N=1  UseFilter=on  TunerSelectOption=Transfer Function Based (PID Tuner App)  InitialConditionSource=internal  InitialConditionForIntegrator=0  InitialConditionForFilter=0  DifferentiatorICPrevScaledInput=0  ExternalReset=either  TrackingMode=off  Kt=1  LimitOutput=off  SatLimitsSource=internal  UpperSaturationLimit=inf  LowerSaturationLimit=-inf  LinearizeAsGain=on  AntiWindupMode=back-calculation  Kb=1  LimitIntegrator=off  UpperIntegratorSaturationLimit=inf  LowerIntegratorSaturationLimit=-inf  POutMin=[]  POutMax=[]  IOutMin=[]  IOutMax=[]  DOutMin=[]  DOutMax=[]  NOutMin=[]  NOutMax=[]  SumOutMin=[]  SumOutMax=[]  SaturationOutMin=[]  SaturationOutMax=[]  PParamMin=[]  PParamMax=[]  IParamMin=[]  IParamMax=[]  DParamMin=[]  DParamMax=[]  NParamMin=[]  NParamMax=[]  KbParamMin=[]  KbParamMax=[]  KtParamMin=[]  KtParamMax=[]  KbOutMin=[]  KbOutMax=[]  KtOutMin=[]  KtOutMax=[]  IntegratorOutMin=[]  IntegratorOutMax=[]  FilterOutMin=[]  FilterOutMax=[]  SumI1OutMin=[]  SumI1OutMax=[]  SumI2OutMin=[]  SumI2OutMax=[]  SumI3OutMin=[]  SumI3OutMax=[]  SumI4OutMin=[]  SumI4OutMax=[]  SumDOutMin=[]  SumDOutMax=[]  DifferentiatorOutMin=[]  DifferentiatorOutMax=[]  FilterDiffOutCoefMin=[]  FilterDiffOutCoefMax=[]  ReciprocalOutMin=[]  ReciprocalOutMax=[]  SumDenOutMin=[]  SumDenOutMax=[]  SumNumOutMin=[]  SumNumOutMax=[]  DivideOutMin=[]  DivideOutMax=[]  UdiffTsProdOutMin=[]  UdiffTsProdOutMax=[]  NTsProdOutMin=[]  NTsProdOutMax=[]  UintegralTsProdOutMin=[]  UintegralTsProdOutMax=[]  UngainTsProdOutMin=[]  UngainTsProdOutMax=[]  ClampingZeroOutDataTypeStr=Inherit: Inherit via back propagation  ClampingZeroOutMin=[]  ClampingZeroOutMax=[]  FilterDenConstantOutDataTypeStr=Inherit: Inherit via back propagation  FilterDenConstantOutMin=[]  FilterDenConstantOutMax=[]  PCopyOutDataTypeStr=Inherit: Inherit via back propagation  PCopyOutMin=[]  PCopyOutMax=[]  NCopyOutDataTypeStr=Inherit: Inherit via back propagation  NCopyOutMin=[]  NCopyOutMax=[]  IntegratorContinuousStateAttributes=''  IntegratorStateMustResolveToSignalObject=off  IntegratorRTWStateStorageClass=Auto  FilterContinuousStateAttributes=''  FilterStateMustResolveToSignalObject=off  FilterRTWStateStorageClass=Auto  ParallelPVariant=InternalParameters  IdealPVariant=Disabled  IVariant=InternalParameters  DVariant=InternalParameters  IntegratorVariant=Continuous  SatVariant=Disabled  AWVariant=Passthrough  PCopyVariant=Disabled  TRVariant=Disabled  FdbkBlocksVariant=Forward  IdealPFdbkVariant=Disabled  SatFdbkVariant=Disabled  DerivativeFilterVariant=ContFilter  NVariant=InternalParameters  NCopyVariant=Disabled  FilterICVariant=InternalICsFilter  IntegratorICVariant=InternalICs  ExternalResetVariant=ExternalReset  TRSumVariant=Passthrough  SumFdbkVariant=Disabled  SumVariant=Sum_PID  TsampFilterVariant=InternalTs  TsampNgainVariant=Passthrough  TsampIntegralVariant=Disabled_SignalSpec  ExternalSaturationOutDataTypeStr=Inherit: Same as second input  DerivativeSourceVariant=ErrorSignal  PreIntVariant=InternalPreInt
  Transfer Fcn : TransferFcn  Denominator=[0.5 1]
  Transfer Fcn1 : TransferFcn  Denominator=[.001 1]
  Transfer Fcn2 : TransferFcn  Denominator=[.001 1]
  Vehicle Slip Angle Error : Subsystem
  trqL2 : Outport  VectorParamsAs1DForOutWhenUnconnected=off
  trqR2 : Outport  Port=2  VectorParamsAs1DForOutWhenUnconnected=off
  wires:
  Compare To Constant1/1 -> Data Type Conversion/1
  Data Type Conversion/1 -> Transfer Fcn/1
  Max Delta Torque/1 -> Calculate Torque Split/2(max_delta_trq)
  nYaw/1 -> Vehicle Slip Angle Error/3(nYaw)
  Enable/1(Enable) -> Calculate Torque Split/1(enable), PID Controller/2  "Enable"
  Gain1/1 -> Calculate Torque Split/4(tq_l), Calculate Torque Split/5(tq_r)
  rBrake/1 -> Compare To Constant1/1
  Gain6/1 -> trqR2/1
  Vehicle Slip Angle Error/1(Error) -> PID Controller/1
  Calculate Torque Split/1(tq_l_out) -> Gain5/1
  Transfer Fcn/1 -> Calculate Torque Split/7(brk)
  Transfer Fcn2/1 -> Accel Torque Request/2(MotSpdR2)
  trqA2/1 -> Gain1/1
  Calculate Torque Split/2(tq_r_out) -> Gain6/1
  wR2/1 -> Transfer Fcn2/1
  PID Controller/1 -> Calculate Torque Split/6(tq_tv)
  Gain5/1 -> trqL2/1
  aSteerWheel/1 -> Enable/2(aSteerWheel), Vehicle Slip Angle Error/2(aSteerWheel)
  vx/1 -> Enable/1(vx), Vehicle Slip Angle Error/1(vx)
  Accel Torque Request/1(TrqMax) -> Calculate Torque Split/3(max_tq)
  Transfer Fcn1/1 -> Accel Torque Request/1(MotSpdL2)
  wL2/1 -> Transfer Fcn1/1

== system sm_car/Controller/TrqVec 4Motor/Spring Control/Spring Control A1 ==
  mL : Inport
  mR : Inport  Port=2
  Inp : Inport  Port=3
  Hydropneumatic : Subsystem  VariantControl=Hydropneumatic  mask{popup_gas_spring=Stiff}
      mask prompts: popup_gas_spring "Gas Spring"
      mask init: same as sm_car/Controller/Default/Spring Control/Spring Control A1/Hydropneumatic
      mask TypeOptions popup_gas_spring: Stiff | Soft
  None : Subsystem  VariantControl=None
  L : Outport  VectorParamsAs1DForOutWhenUnconnected=off
  R : Outport  Port=2  VectorParamsAs1DForOutWhenUnconnected=off

== system sm_car/Controller/TrqVec 4Motor/Spring Control/Spring Control A2 ==
  mL : Inport
  mR : Inport  Port=2
  Inp : Inport  Port=3
  Hydropneumatic : Subsystem  VariantControl=Hydropneumatic  mask{popup_gas_spring=Stiff}
      mask prompts: popup_gas_spring "Gas Spring"
      mask init: same as sm_car/Controller/Default/Spring Control/Spring Control A1/Hydropneumatic
      mask TypeOptions popup_gas_spring: Stiff | Soft
  None : Subsystem  VariantControl=None
  L : Outport  VectorParamsAs1DForOutWhenUnconnected=off
  R : Outport  Port=2  VectorParamsAs1DForOutWhenUnconnected=off

== system sm_car/Controller/TrqVec 4Motor/Susp/Steer Axle 1 ==
  note: Example Steer by Wire algorithm.
      | Used by steering models where rack position
      | and steering wheel angle inputs are both used.
  aSteerWheel : Inport
  vx : Inport  Port=2
  Bus Creator4 : BusCreator  Inputs=2
  Product1 : Product
  Transfer Fcn (with initial states)1 : simulink_extras/Additional Linear/Transfer Fcn (with initial states)  N=[1]  D="[1/Steer.fActuatorCutoff.Value  1]"  X0=-1
  Vehicle Speed to Ratio Scale : Lookup_n-D  NumberOfTableDimensions=1  BreakpointsForDimension1=Control.Default.Steer.Ratio_Scale.vVehicle.Value  Table=Control.Default.Steer.Ratio_Scale.n.Value  InternalRulePriority=Speed  RndMeth=Simplest
  Wheel Angle to Steer Ratio : Lookup_n-D  NumberOfTableDimensions=1  BreakpointsForDimension1=Control.Default.Steer.Ratio_Table.aWheel.Value  Table=Control.Default.Steer.Ratio_Table.xRack.Value  InternalRulePriority=Speed  RndMeth=Simplest
  Steer : Outport  VectorParamsAs1DForOutWhenUnconnected=off
  wires:
  Vehicle Speed to Ratio Scale/1 -> Product1/1  "nRatioScale"
  Transfer Fcn (with initial states)1/1 -> Vehicle Speed to Ratio Scale/1
  aSteerWheel/1 -> Wheel Angle to Steer Ratio/1, Bus Creator4/2  "aSteerWheel"
  Wheel Angle to Steer Ratio/1 -> Product1/2  "xRack"
  Product1/1 -> Bus Creator4/1  "xRack"
  vx/1 -> Transfer Fcn (with initial states)1/1
  Bus Creator4/1 -> Steer/1  "Steer"

== system sm_car/Controller/TrqVec 4Motor/Susp/Steer Axle 2 ==
  note: Example rear steer algorithm
      | Rack position is based on steering wheel angle
      | and is scaled based on vehicle speed.
  aSteerWheel : Inport
  vx : Inport  Port=2
  1-D Lookup Table : Lookup_n-D  NumberOfTableDimensions=1  BreakpointsForDimension1=Steer.Gain.vVehicle.Value  Table=Steer.Gain.n.Value  InterpMethod=Linear Lagrange  InternalRulePriority=Speed  RndMeth=Simplest
  Bus Creator2 : BusCreator  Inputs=2
  Filter : simulink_extras/Additional Linear/Transfer Fcn (with initial states)  N=[1]  D="[1/Steer.fActuatorCutoff.Value  1]"  X0=-1
  Gain : Gain  Gain=3.6
  Gain1 : Gain  Gain=Steer.Gain.nRearAct.Value
  Product : Product
  Saturation : Saturate  UpperLimit=Steer.Limits.aUpper.Value  LowerLimit=Steer.Limits.aLower.Value  LinearizeAsGain=off  ZeroCross=off
  Steer : Outport
  wires:
  aSteerWheel/1 -> Product/1
  Gain/1 -> 1-D Lookup Table/1
  Bus Creator2/1 -> Steer/1  "Steer"
  Saturation/1 -> Bus Creator2/1, Gain1/1  "aSteerWheel"
  Product/1 -> Saturation/1
  Filter/1 -> Product/2
  Gain1/1 -> Bus Creator2/2  "xSteerActuator"
  1-D Lookup Table/1 -> Filter/1
  vx/1 -> Gain/1

== system sm_car/Driver/Closed Loop/Driver/Cur Pose ==
  Cur : Inport
  Demux : Demux  Outputs=3
  Gain : Gain  Gain=pi/180
  Mux : Mux  Inputs=3
  CurPose : Outport  VectorParamsAs1DForOutWhenUnconnected=off
  wires:
  Gain/1 -> Mux/3
  Demux/3 -> Gain/1
  Demux/2 -> Mux/2
  Mux/1 -> CurPose/1
  Cur/1 -> Demux/1
  Demux/1 -> Mux/1

== system sm_car/Driver/Closed Loop/Driver/Fwd Rev ==
  note: This logic enables the driver models to handle maneuvers where the vehicle is driven in reverse.
  note: When driving in reverse, swap sign so that only positive velocities are fed to Longitudinal Driver model.
  vx : Inport
  vT : Inport  Port=2
  Product : Product
  Sign : Signum  ZeroCross=off
  dir : Outport
  vxFwRv : Outport  Port=2
  wires:
  Product/1 -> vxFwRv/1
  vx/1 -> Product/1
  Sign/1 -> Product/2, dir/1  "Direction"
  vT/1 -> Sign/1

== system sm_car/Driver/Closed Loop/Driver/Lateral Driver ==
  referencePose : Inport
  Distance : Inport  Port=2
  currentPose : Inport  Port=3
  v_x : Inport  Port=4
  Preview : Inport  Port=5
  Direction : Inport  Port=6
  Pure Pursuit : Subsystem  VariantControl=Pure_Pursuit  mask(Lateral Driver (Pure Pursuit)){MAX_STEERING_ANGLE_DEG=Lateral.aMaxSteer.Value, L_AXLE_DIST=Lateral.xWheelbase.Value, LOOKAHEAD_GAIN_KPP=Lateral.Pursuit.kLookahead.Value, MIN_LOOKAHEAD_DIST=Lateral.Pursuit.xLookaheadMin.Value, MAX_LOOKAHEAD_DIST=Lateral.Pursuit.xLookaheadMax.Value, HEADING_WEIGHT_KH=Lateral.Pursuit.nWeightHeadingErr.Value}
      mask prompts: MAX_STEERING_ANGLE_DEG "Maximum steering angle (degrees)"; L_AXLE_DIST "Distance from the vehicle's reference point (currentPose) to the front axle (m)"; LOOKAHEAD_GAIN_KPP "Proportional gain for lookahead distance (Ld = K_pp * v_x)"; MIN_LOOKAHEAD_DIST "Minimum lookahead distance (m)"; MAX_LOOKAHEAD_DIST "Maximum lookahead distance (m)"; HEADING_WEIGHT_KH "Weight for the heading error term"
      mask help:
      | Implements PurePursuit method for lateral control.
      | Supports forward and reverse driving.
      | Pure Pursuit is based on Coulter, R. Craig. (1992). Implementation of the Pure Pursuit Path Tracking Algorithm. Carnegie Mellon University, The Robotics Institute. Technical Report CMU-RI-TR-92-01.
      mask DialogControl Container5 Prompt: Vehicle Parameters
      mask DialogControl Container4 Prompt: Pure Pursuit Method Parameters
  Stanley : Subsystem  VariantControl=Stanley  mask(Lateral Driver (Stanley)){MAX_STEERING_ANGLE_DEG=Lateral.aMaxSteer.Value, L_AXLE_DIST=Lateral.xWheelbase.Value, K_cte_forward=Lateral.Stanley.NForward.Value, K_cte_reverse=Lateral.Stanley.NReverse.Value}
      mask prompts: MAX_STEERING_ANGLE_DEG "Maximum steering angle (degrees)"; L_AXLE_DIST "Distance from the vehicle's reference point (currentPose) to the front axle (m)"; K_cte_forward "Cross-track error gain for forward"; K_cte_reverse "Cross-track error gain for reverse"
      mask help:
      | Implements Stanley method for lateral control.
      | Supports forward and reverse driving.
      | Stanley method is based on Hoffmann et al. (2007), "Autonomous Automobile Trajectory Tracking for Off-Road Driving"
      mask DialogControl Container5 Prompt: Vehicle Parameters
      mask DialogControl Container3 Prompt: Stanley Method Parameters
  steeringAngle : Outport
